simulink model "SimulinkModell"  (R2017b)
settings: Solver=VariableStepAuto  StartTime=0.0  StopTime=10.0  RelTol=1e-3
settings Model: Creator=Lucas  LastModifiedBy=Lucas

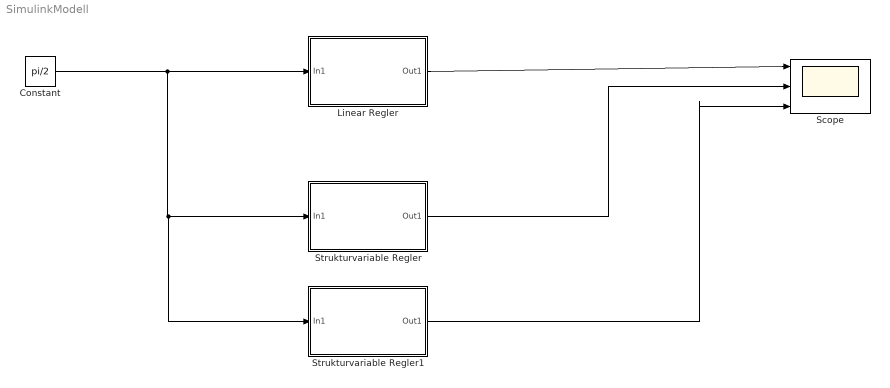
== system SimulinkModell ==
  Constant : Constant  Value=pi/2
  Linear Regler : Subsystem
  Scope : Scope  NumInputPorts=3
  Strukturvariable Regler : Subsystem
  Strukturvariable Regler1 : Subsystem
  wires:
  Constant/1 -> Strukturvariable Regler1/1(In1), Strukturvariable Regler/1(In1), Linear Regler/1(In1)
  Linear Regler/1(Out1) -> Scope/1
  Strukturvariable Regler/1(Out1) -> Scope/2
  Strukturvariable Regler1/1(Out1) -> Scope/3

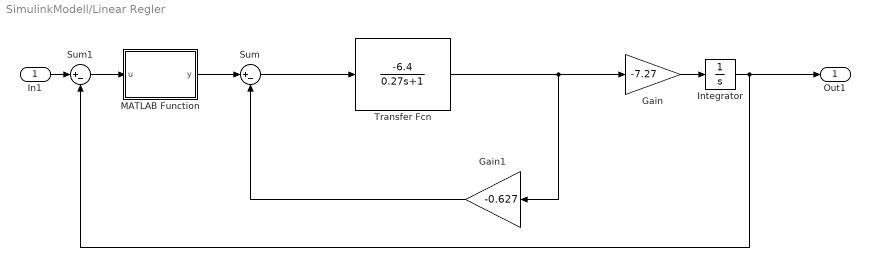
== system SimulinkModell/Linear Regler ==
  In1 : Inport
  Gain : Gain  Gain=-7.27
  Gain1 : Gain  Gain=-0.627
  Integrator : Integrator  InitialCondition=pi/3
  MATLAB Function : MATLAB Function  TreatAsAtomicUnit=on
  Sum : Sum  Inputs=|+-
  Sum1 : Sum  Inputs=|+-
  Transfer Fcn : TransferFcn  Numerator=[-6.4]  Denominator=[0.27 1]
  Out1 : Outport
  wires:
  Gain1/1 -> Sum/2
  Transfer Fcn/1 -> Gain1/1, Gain/1
  Gain/1 -> Integrator/1
  In1/1 -> Sum1/1
  Integrator/1 -> Out1/1, Sum1/2
  Sum1/1 -> MATLAB Function/1(u)
  MATLAB Function/1(y) -> Sum/1
  Sum/1 -> Transfer Fcn/1

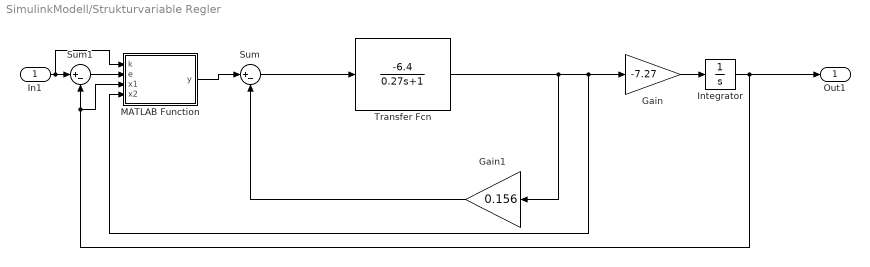
== system SimulinkModell/Strukturvariable Regler ==
  In1 : Inport
  Gain : Gain  Gain=-7.27
  Gain1 : Gain  Gain=0.156
  Integrator : Integrator  InitialCondition=pi/3
  MATLAB Function : MATLAB Function  TreatAsAtomicUnit=on
  Sum : Sum  Inputs=|+-
  Sum1 : Sum  Inputs=|+-
  Transfer Fcn : TransferFcn  Numerator=[-6.4]  Denominator=[0.27 1]
  Out1 : Outport
  wires:
  Gain1/1 -> Sum/2
  Transfer Fcn/1 -> Gain1/1, MATLAB Function/4(x2), Gain/1
  Gain/1 -> Integrator/1
  In1/1 -> MATLAB Function/1(k), Sum1/1
  Integrator/1 -> Out1/1, MATLAB Function/3(x1), Sum1/2
  MATLAB Function/1(y) -> Sum/1
  Sum/1 -> Transfer Fcn/1
  Sum1/1 -> MATLAB Function/2(e)

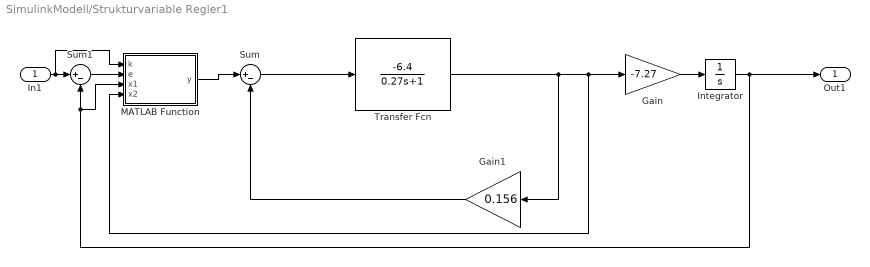
== system SimulinkModell/Strukturvariable Regler1 ==
  In1 : Inport
  Gain : Gain  Gain=-7.27
  Gain1 : Gain  Gain=0.156
  Integrator : Integrator  InitialCondition=pi/3
  MATLAB Function : MATLAB Function  TreatAsAtomicUnit=on
  Sum : Sum  Inputs=|+-
  Sum1 : Sum  Inputs=|+-
  Transfer Fcn : TransferFcn  Numerator=[-6.4]  Denominator=[0.27 1]
  Out1 : Outport
  wires:
  Sum1/1 -> MATLAB Function/2(e)
  Sum/1 -> Transfer Fcn/1
  MATLAB Function/1(y) -> Sum/1
  Integrator/1 -> Sum1/2, MATLAB Function/3(x1), Out1/1
  In1/1 -> Sum1/1, MATLAB Function/1(k)
  Gain/1 -> Integrator/1
  Transfer Fcn/1 -> Gain/1, MATLAB Function/4(x2), Gain1/1
  Gain1/1 -> Sum/2

== matlab function SimulinkModell/Strukturvariable Regler/MATLAB Function ==
  data: k input; e input; x1 input; y output; x2 input
function y = fcn(k, e, x1, x2)
aux = 0;
if(x2*(x1-k)) > 0
    aux = 0.1*e;
elseif (x2*(x1-k)) <= 0
    aux = 0.5*e;
end
y = aux;

== matlab function SimulinkModell/Linear Regler/MATLAB Function ==
  data: u input; y output
function y = fcn(u)

y = 0.5*u;

== matlab function SimulinkModell/Strukturvariable Regler1/MATLAB Function ==
  data: k input; e input; x1 input; y output; x2 input
function y = fcn(k, e, x1, x2)
aux = 0;
if(x2*(x1-k)) > 0
    aux = 0.1*e;
elseif (x2*(x1-k)) <= 0
    aux = 0.5*e;
end
y = aux;
